simulink model "LQR"  (R2023a)
settings: Solver=VariableStepAuto  StartTime=0.0  StopTime=10  RelTol=1e-3
values from neighbouring files (symbols this model uses):
  A = [0.99 0.03 -0.02 -0.32 ... (first row only)    [HewersAlgorithm.m]
  B = [0.01 0.88 ... (first row only)    [HewersAlgorithm.m]
  F0 = inv(R+B'*Pi*B)*B'*Pi*A    [HewersAlgorithm.m]
  x0 = [1; 1; 1; 1]    [HewersAlgorithm.m]
settings Model: Creator=pavandattareddy  LastModifiedBy=pavandattareddy
settings DebuggingCC: AlgebraicLoopMsg=none

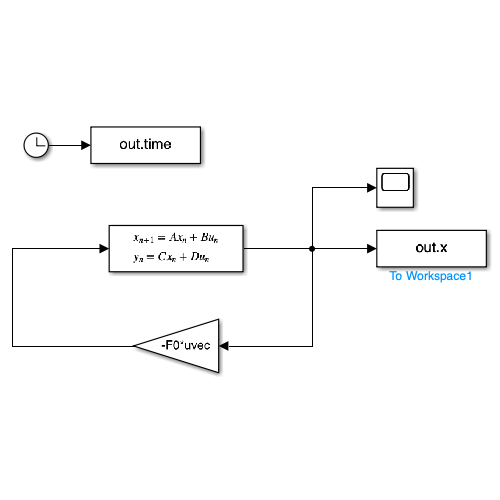
[thumbnail: Simulink's stored preview of the top-level diagram]
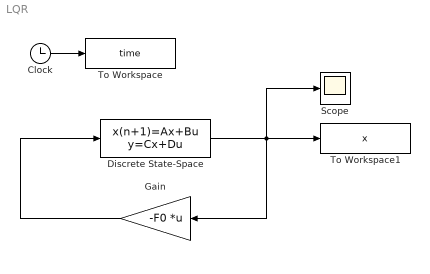
== system LQR ==
  Clock : Clock
  Discrete State-Space : DiscreteStateSpace  A=A  B=B  C=A  D=B  InitialCondition=x0  SampleTime=-1
  Gain : Gain  Gain=-F0  Multiplication=Matrix(K*u) (u vector)
  Scope : Scope
  To Workspace : ToWorkspace  VariableName=time  SaveFormat=Timeseries  SampleTime=-1
  To Workspace1 : ToWorkspace  VariableName=x  SaveFormat=Timeseries  SampleTime=-1
  wires:
  Discrete State-Space/1 -> Gain/1, To Workspace1/1, Scope/1
  Gain/1 -> Discrete State-Space/1
  Clock/1 -> To Workspace/1
